simulink library "ECO_TestLibs"  (R2018a)
settings: Solver=ode45  StartTime=0.0  StopTime=10.0  RelTol=1e-3  EnableMultiTasking=on
undefined symbols (not defined in the file or in its folder): h, km
libraries: CoderSF_BSW_Libs x643, $bdroot x217, SF_CanService_Libs x60, simulink x12
(part 4 of 7)

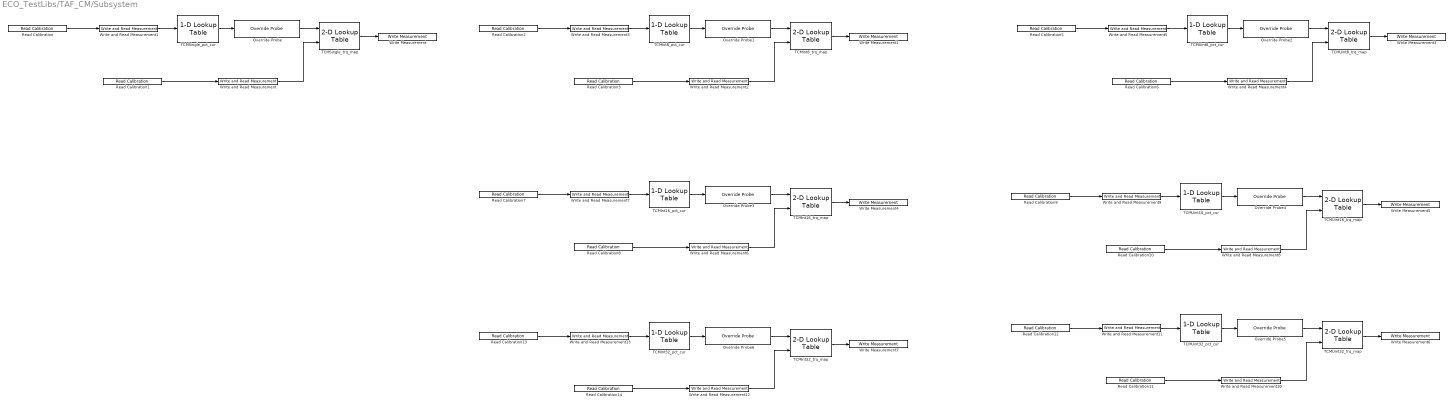
== system ECO_TestLibs/TAF_CM/Subsystem ==
  " Override Probe" : CoderSF_BSW_Libs/Calibration & Measurement/ Override Probe  variableName=TCMSingle_pct  variableValue=9  overrideValue=0  variableDataType=single  variableMin=[]  variableMax=[]  variableUnitStr=%
      settings: SourceProductName=EcoCoder Blocks
  " Override Probe1" : CoderSF_BSW_Libs/Calibration & Measurement/ Override Probe  variableName=TCMInt8_pct  variableValue=9  overrideValue=0  variableDataType=int8  variableMin=[]  variableMax=[]  variableUnitStr=%
      settings: SourceProductName=EcoCoder Blocks
  " Override Probe2" : CoderSF_BSW_Libs/Calibration & Measurement/ Override Probe  variableName=TCMUint8_pct  variableValue=9  overrideValue=0  variableDataType=uint8  variableMin=[]  variableMax=[]  variableUnitStr=%
      settings: SourceProductName=EcoCoder Blocks
  " Override Probe3" : CoderSF_BSW_Libs/Calibration & Measurement/ Override Probe  variableName=TCMInt16_pct  variableValue=9  overrideValue=0  variableDataType=int16  variableMin=[]  variableMax=[]  variableUnitStr=%
      settings: SourceProductName=EcoCoder Blocks
  " Override Probe4" : CoderSF_BSW_Libs/Calibration & Measurement/ Override Probe  variableName=TCMUint16_pct  variableValue=9  overrideValue=0  variableDataType=uint16  variableMin=[]  variableMax=[]  variableUnitStr=%
      settings: SourceProductName=EcoCoder Blocks
  " Override Probe5" : CoderSF_BSW_Libs/Calibration & Measurement/ Override Probe  variableName=TCMUint32_pct  variableValue=9  overrideValue=0  variableDataType=uint32  variableMin=[]  variableMax=[]  variableUnitStr=%
      settings: SourceProductName=EcoCoder Blocks
  " Override Probe6" : CoderSF_BSW_Libs/Calibration & Measurement/ Override Probe  variableName=TCMInt32_pct  variableValue=9  overrideValue=0  variableDataType=int32  variableMin=[]  variableMax=[]  variableUnitStr=%
      settings: SourceProductName=EcoCoder Blocks
  Read Calibration : CoderSF_BSW_Libs/Calibration & Measurement/Read Calibration  variable_name=TCMSingle_volt_val  variable_value=1  variable_type=single  variable_min=[]  variable_max=[]  unitStr=V  descStr=""
      settings: AttributesFormatString=value:%<variable_value> type:%<variable_type> max:%<variable_max> Min:%<variable_min>  SourceProductName=EcoCoder Blocks
  Read Calibration1 : CoderSF_BSW_Libs/Calibration & Measurement/Read Calibration  variable_name=TCMSingle_linspd_val  variable_value=20  variable_type=single  variable_min=[]  variable_max=[]  unitStr=km/h  descStr=""
      settings: AttributesFormatString=value:%<variable_value> type:%<variable_type> max:%<variable_max> Min:%<variable_min>  SourceProductName=EcoCoder Blocks
  Read Calibration10 : CoderSF_BSW_Libs/Calibration & Measurement/Read Calibration  variable_name=TCMUint16_linspd_val  variable_value=20  variable_type=uint16  variable_min=[]  variable_max=[]  unitStr=km/h  descStr=""
      settings: AttributesFormatString=value:%<variable_value> type:%<variable_type> max:%<variable_max> Min:%<variable_min>  SourceProductName=EcoCoder Blocks
  Read Calibration11 : CoderSF_BSW_Libs/Calibration & Measurement/Read Calibration  variable_name=TCMUint32_linspd_val  variable_value=20  variable_type=uint32  variable_min=[]  variable_max=[]  unitStr=km/h  descStr=""
      settings: AttributesFormatString=value:%<variable_value> type:%<variable_type> max:%<variable_max> Min:%<variable_min>  SourceProductName=EcoCoder Blocks
  Read Calibration12 : CoderSF_BSW_Libs/Calibration & Measurement/Read Calibration  variable_name=TCMUint32_volt_val  variable_value=1  variable_type=uint32  variable_min=[]  variable_max=[]  unitStr=V  descStr=""
      settings: AttributesFormatString=value:%<variable_value> type:%<variable_type> max:%<variable_max> Min:%<variable_min>  SourceProductName=EcoCoder Blocks
  Read Calibration13 : CoderSF_BSW_Libs/Calibration & Measurement/Read Calibration  variable_name=TCMInt32_volt_val  variable_value=1  variable_type=int32  variable_min=[]  variable_max=[]  unitStr=V  descStr=""
      settings: AttributesFormatString=value:%<variable_value> type:%<variable_type> max:%<variable_max> Min:%<variable_min>  SourceProductName=EcoCoder Blocks
  Read Calibration14 : CoderSF_BSW_Libs/Calibration & Measurement/Read Calibration  variable_name=TCMInt32_linspd_val  variable_value=20  variable_type=int32  variable_min=[]  variable_max=[]  unitStr=km/h  descStr=""
      settings: AttributesFormatString=value:%<variable_value> type:%<variable_type> max:%<variable_max> Min:%<variable_min>  SourceProductName=EcoCoder Blocks
  Read Calibration2 : CoderSF_BSW_Libs/Calibration & Measurement/Read Calibration  variable_name=TCMInt8_volt_val  variable_value=1  variable_type=int8  variable_min=[]  variable_max=[]  unitStr=V  descStr=""
      settings: AttributesFormatString=value:%<variable_value> type:%<variable_type> max:%<variable_max> Min:%<variable_min>  SourceProductName=EcoCoder Blocks
  Read Calibration3 : CoderSF_BSW_Libs/Calibration & Measurement/Read Calibration  variable_name=TCMInt8_linspd_val  variable_value=20  variable_type=int8  variable_min=[]  variable_max=[]  unitStr=km/h  descStr=""
      settings: AttributesFormatString=value:%<variable_value> type:%<variable_type> max:%<variable_max> Min:%<variable_min>  SourceProductName=EcoCoder Blocks
  Read Calibration5 : CoderSF_BSW_Libs/Calibration & Measurement/Read Calibration  variable_name=TCMUint8_volt_val  variable_value=1  variable_type=uint8  variable_min=[]  variable_max=[]  unitStr=V  descStr=""
      settings: AttributesFormatString=value:%<variable_value> type:%<variable_type> max:%<variable_max> Min:%<variable_min>  SourceProductName=EcoCoder Blocks
  Read Calibration6 : CoderSF_BSW_Libs/Calibration & Measurement/Read Calibration  variable_name=TCMUint8_linspd_val  variable_value=20  variable_type=uint8  variable_min=[]  variable_max=[]  unitStr=km/h  descStr=""
      settings: AttributesFormatString=value:%<variable_value> type:%<variable_type> max:%<variable_max> Min:%<variable_min>  SourceProductName=EcoCoder Blocks
  Read Calibration7 : CoderSF_BSW_Libs/Calibration & Measurement/Read Calibration  variable_name=TCMInt16_volt_val  variable_value=1  variable_type=int16  variable_min=[]  variable_max=[]  unitStr=V  descStr=""
      settings: AttributesFormatString=value:%<variable_value> type:%<variable_type> max:%<variable_max> Min:%<variable_min>  SourceProductName=EcoCoder Blocks
  Read Calibration8 : CoderSF_BSW_Libs/Calibration & Measurement/Read Calibration  variable_name=TCMInt16_linspd_val  variable_value=20  variable_type=int16  variable_min=[]  variable_max=[]  unitStr=km/h  descStr=""
      settings: AttributesFormatString=value:%<variable_value> type:%<variable_type> max:%<variable_max> Min:%<variable_min>  SourceProductName=EcoCoder Blocks
  Read Calibration9 : CoderSF_BSW_Libs/Calibration & Measurement/Read Calibration  variable_name=TCMUint16_volt_val  variable_value=1  variable_type=uint16  variable_min=[]  variable_max=[]  unitStr=V  descStr=""
      settings: AttributesFormatString=value:%<variable_value> type:%<variable_type> max:%<variable_max> Min:%<variable_min>  SourceProductName=EcoCoder Blocks
  TCMInt16_pct_cur : CoderSF_BSW_Libs/Calibration & Measurement/1-D Lookup Table  nam=TCMInt16_pct  breakpoint_type=int16  breakpoint_data=[0 5]  table_type=int16  table_data=[0 100]
      settings: SourceProductName=EcoCoder Blocks
  TCMInt16_trq_map : CoderSF_BSW_Libs/Calibration & Measurement/2-D Lookup Table  nam=TCMInt16_trq  breakpoint1_type=int16  breakpoint1_data=[0 50 100]  breakpoint2_type=int16  breakpoint2_data=[0 40 80 120]  table_type=int16  table_data=[20 40 40 30 ;20 50 40 30;20 40 50 80]
      settings: SourceProductName=EcoCoder Blocks
  TCMInt32_pct_cur : CoderSF_BSW_Libs/Calibration & Measurement/1-D Lookup Table  nam=TCMInt32_pct  breakpoint_type=int32  breakpoint_data=[0 5]  table_type=int32  table_data=[0 100]
      settings: SourceProductName=EcoCoder Blocks
  TCMInt32_trq_map : CoderSF_BSW_Libs/Calibration & Measurement/2-D Lookup Table  nam=TCMInt32_trq  breakpoint1_type=int32  breakpoint1_data=[0 50 100]  breakpoint2_type=int32  breakpoint2_data=[0 40 80 120]  table_type=int32  table_data=[20 40 40 30 ;20 50 40 30;20 40 50 80]
      settings: SourceProductName=EcoCoder Blocks
  TCMInt8_pct_cur : CoderSF_BSW_Libs/Calibration & Measurement/1-D Lookup Table  nam=TCMInt8_pct  breakpoint_type=int8  breakpoint_data=[0 5]  table_type=int8  table_data=[0 100]
      settings: SourceProductName=EcoCoder Blocks
  TCMInt8_trq_map : CoderSF_BSW_Libs/Calibration & Measurement/2-D Lookup Table  nam=TCMInt8_trq  breakpoint1_type=int8  breakpoint1_data=[0 50 100]  breakpoint2_type=int8  breakpoint2_data=[0 40 80 120]  table_type=int8  table_data=[20 40 40 30 ;20 50 40 30;20 40 50 80]
      settings: SourceProductName=EcoCoder Blocks
  TCMSingle_pct_cur : CoderSF_BSW_Libs/Calibration & Measurement/1-D Lookup Table  nam=TCMSingle_pct  breakpoint_type=single  breakpoint_data=[0 5]  table_type=single  table_data=[0 100]
      settings: SourceProductName=EcoCoder Blocks
  TCMSingle_trq_map : CoderSF_BSW_Libs/Calibration & Measurement/2-D Lookup Table  nam=TCMSingle_trq  breakpoint1_type=single  breakpoint1_data=[0 50 100]  breakpoint2_type=single  breakpoint2_data=[0 40 80 120]  table_type=single  table_data=[20 40 40 30 ;20 50 40 30;20 40 50 80]
      settings: SourceProductName=EcoCoder Blocks
  TCMUint16_pct_cur : CoderSF_BSW_Libs/Calibration & Measurement/1-D Lookup Table  nam=TCMUint16_pct  breakpoint_type=uint16  breakpoint_data=[0 5]  table_type=uint16  table_data=[0 100]
      settings: SourceProductName=EcoCoder Blocks
  TCMUint16_trq_map : CoderSF_BSW_Libs/Calibration & Measurement/2-D Lookup Table  nam=TCMUint16_trq  breakpoint1_type=uint16  breakpoint1_data=[0 50 100]  breakpoint2_type=uint16  breakpoint2_data=[0 40 80 120]  table_type=uint16  table_data=[20 40 40 30 ;20 50 40 30;20 40 50 80]
      settings: SourceProductName=EcoCoder Blocks
  TCMUint32_pct_cur : CoderSF_BSW_Libs/Calibration & Measurement/1-D Lookup Table  nam=TCMUint32_pct  breakpoint_type=uint32  breakpoint_data=[0 5]  table_type=uint32  table_data=[0 100]
      settings: SourceProductName=EcoCoder Blocks
  TCMUint32_trq_map : CoderSF_BSW_Libs/Calibration & Measurement/2-D Lookup Table  nam=TCMUint32_trq  breakpoint1_type=uint32  breakpoint1_data=[0 50 100]  breakpoint2_type=uint32  breakpoint2_data=[0 40 80 120]  table_type=uint32  table_data=[20 40 40 30 ;20 50 40 30;20 40 50 80]
      settings: SourceProductName=EcoCoder Blocks
  TCMUint8_pct_cur : CoderSF_BSW_Libs/Calibration & Measurement/1-D Lookup Table  nam=TCMUint8_pct  breakpoint_type=uint8  breakpoint_data=[0 5]  table_type=uint8  table_data=[0 100]
      settings: SourceProductName=EcoCoder Blocks
  TCMUint8_trq_map : CoderSF_BSW_Libs/Calibration & Measurement/2-D Lookup Table  nam=TCMUint8_trq  breakpoint1_type=uint8  breakpoint1_data=[0 50 100]  breakpoint2_type=uint8  breakpoint2_data=[0 40 80 120]  table_type=uint8  table_data=[20 40 40 30 ;20 50 40 30;20 40 50 80]
      settings: SourceProductName=EcoCoder Blocks
  Write Measurement : CoderSF_BSW_Libs/Calibration & Measurement/Write Measurement  variable_name=TCMSingle_trq  variable_value=0  variable_type=single  numD=1  unitStr=Nm  descStr=""
      settings: AttributesFormatString=value:%<variable_value> type:%<variable_type>  SourceProductName=EcoCoder Blocks
  Write Measurement1 : CoderSF_BSW_Libs/Calibration & Measurement/Write Measurement  variable_name=TCMInt8_trq  variable_value=0  variable_type=int8  numD=1  unitStr=Nm  descStr=""
      settings: AttributesFormatString=value:%<variable_value> type:%<variable_type>  SourceProductName=EcoCoder Blocks
  Write Measurement3 : CoderSF_BSW_Libs/Calibration & Measurement/Write Measurement  variable_name=TCMUint8_trq  variable_value=0  variable_type=uint8  numD=1  unitStr=Nm  descStr=""
      settings: AttributesFormatString=value:%<variable_value> type:%<variable_type>  SourceProductName=EcoCoder Blocks
  Write Measurement4 : CoderSF_BSW_Libs/Calibration & Measurement/Write Measurement  variable_name=TCMInt16_trq  variable_value=0  variable_type=int16  numD=1  unitStr=Nm  descStr=""
      settings: AttributesFormatString=value:%<variable_value> type:%<variable_type>  SourceProductName=EcoCoder Blocks
  Write Measurement5 : CoderSF_BSW_Libs/Calibration & Measurement/Write Measurement  variable_name=TCMUint16_trq  variable_value=0  variable_type=uint16  numD=1  unitStr=Nm  descStr=""
      settings: AttributesFormatString=value:%<variable_value> type:%<variable_type>  SourceProductName=EcoCoder Blocks
  Write Measurement6 : CoderSF_BSW_Libs/Calibration & Measurement/Write Measurement  variable_name=TCMUint32_trq  variable_value=0  variable_type=uint32  numD=1  unitStr=Nm  descStr=""
      settings: AttributesFormatString=value:%<variable_value> type:%<variable_type>  SourceProductName=EcoCoder Blocks
  Write Measurement7 : CoderSF_BSW_Libs/Calibration & Measurement/Write Measurement  variable_name=TCMInt32_trq  variable_value=0  variable_type=int32  numD=1  unitStr=Nm  descStr=""
      settings: AttributesFormatString=value:%<variable_value> type:%<variable_type>  SourceProductName=EcoCoder Blocks
  Write and Read Measurement : CoderSF_BSW_Libs/Calibration & Measurement/Write and Read Measurement  variable_name=TCMSingle_linspd  variable_value=0  variable_type=single  numD=1  unitStr=km/h  descStr=""
      settings: AttributesFormatString=value:%<variable_value> type:%<variable_type>  SourceProductName=EcoCoder Blocks
  Write and Read Measurement1 : CoderSF_BSW_Libs/Calibration & Measurement/Write and Read Measurement  variable_name=TCMSingle_volt  variable_value=0  variable_type=single  numD=1  unitStr=V  descStr=""
      settings: AttributesFormatString=value:%<variable_value> type:%<variable_type>  SourceProductName=EcoCoder Blocks
  Write and Read Measurement10 : CoderSF_BSW_Libs/Calibration & Measurement/Write and Read Measurement  variable_name=TCMUint32_linspd  variable_value=0  variable_type=uint32  numD=1  unitStr=km/h  descStr=""
      settings: AttributesFormatString=value:%<variable_value> type:%<variable_type>  SourceProductName=EcoCoder Blocks
  Write and Read Measurement11 : CoderSF_BSW_Libs/Calibration & Measurement/Write and Read Measurement  variable_name=TCMUint32_volt  variable_value=0  variable_type=uint32  numD=1  unitStr=V  descStr=""
      settings: AttributesFormatString=value:%<variable_value> type:%<variable_type>  SourceProductName=EcoCoder Blocks
  Write and Read Measurement12 : CoderSF_BSW_Libs/Calibration & Measurement/Write and Read Measurement  variable_name=TCMInt32_linspd  variable_value=0  variable_type=int32  numD=1  unitStr=km/h  descStr=""
      settings: AttributesFormatString=value:%<variable_value> type:%<variable_type>  SourceProductName=EcoCoder Blocks
  Write and Read Measurement13 : CoderSF_BSW_Libs/Calibration & Measurement/Write and Read Measurement  variable_name=TCMInt32_volt  variable_value=0  variable_type=int32  numD=1  unitStr=V  descStr=""
      settings: AttributesFormatString=value:%<variable_value> type:%<variable_type>  SourceProductName=EcoCoder Blocks
  Write and Read Measurement2 : CoderSF_BSW_Libs/Calibration & Measurement/Write and Read Measurement  variable_name=TCMInt8_linspd  variable_value=0  variable_type=int8  numD=1  unitStr=km/h  descStr=""
      settings: AttributesFormatString=value:%<variable_value> type:%<variable_type>  SourceProductName=EcoCoder Blocks
  Write and Read Measurement3 : CoderSF_BSW_Libs/Calibration & Measurement/Write and Read Measurement  variable_name=TCMInt8_volt  variable_value=0  variable_type=int8  numD=1  unitStr=V  descStr=""
      settings: AttributesFormatString=value:%<variable_value> type:%<variable_type>  SourceProductName=EcoCoder Blocks
  Write and Read Measurement4 : CoderSF_BSW_Libs/Calibration & Measurement/Write and Read Measurement  variable_name=TCMUint8_linspd  variable_value=0  variable_type=uint8  numD=1  unitStr=km/h  descStr=""
      settings: AttributesFormatString=value:%<variable_value> type:%<variable_type>  SourceProductName=EcoCoder Blocks
  Write and Read Measurement5 : CoderSF_BSW_Libs/Calibration & Measurement/Write and Read Measurement  variable_name=TCMUint8_volt  variable_value=0  variable_type=uint8  numD=1  unitStr=V  descStr=""
      settings: AttributesFormatString=value:%<variable_value> type:%<variable_type>  SourceProductName=EcoCoder Blocks
  Write and Read Measurement6 : CoderSF_BSW_Libs/Calibration & Measurement/Write and Read Measurement  variable_name=TCMInt16_linspd  variable_value=0  variable_type=int16  numD=1  unitStr=km/h  descStr=""
      settings: AttributesFormatString=value:%<variable_value> type:%<variable_type>  SourceProductName=EcoCoder Blocks
  Write and Read Measurement7 : CoderSF_BSW_Libs/Calibration & Measurement/Write and Read Measurement  variable_name=TCMInt16_volt  variable_value=0  variable_type=int16  numD=1  unitStr=V  descStr=""
      settings: AttributesFormatString=value:%<variable_value> type:%<variable_type>  SourceProductName=EcoCoder Blocks
  Write and Read Measurement8 : CoderSF_BSW_Libs/Calibration & Measurement/Write and Read Measurement  variable_name=TCMUint16_linspd  variable_value=0  variable_type=uint16  numD=1  unitStr=km/h  descStr=""
      settings: AttributesFormatString=value:%<variable_value> type:%<variable_type>  SourceProductName=EcoCoder Blocks
  Write and Read Measurement9 : CoderSF_BSW_Libs/Calibration & Measurement/Write and Read Measurement  variable_name=TCMUint16_volt  variable_value=0  variable_type=uint16  numD=1  unitStr=V  descStr=""
      settings: AttributesFormatString=value:%<variable_value> type:%<variable_type>  SourceProductName=EcoCoder Blocks
  wires:
  Read Calibration12/1 -> Write and Read Measurement11/1
  TCMUint32_pct_cur/1 -> " Override Probe5"/1
  Read Calibration/1 -> Write and Read Measurement1/1
  " Override Probe"/1 -> TCMSingle_trq_map/1
  TCMSingle_pct_cur/1 -> " Override Probe"/1
  Write and Read Measurement/1 -> TCMSingle_trq_map/2
  Write and Read Measurement1/1 -> TCMSingle_pct_cur/1
  TCMSingle_trq_map/1 -> Write Measurement/1
  Read Calibration1/1 -> Write and Read Measurement/1
  Read Calibration2/1 -> Write and Read Measurement3/1
  TCMInt8_pct_cur/1 -> " Override Probe1"/1
  " Override Probe1"/1 -> TCMInt8_trq_map/1
  Write and Read Measurement2/1 -> TCMInt8_trq_map/2
  Read Calibration3/1 -> Write and Read Measurement2/1
  TCMInt8_trq_map/1 -> Write Measurement1/1
  Write and Read Measurement3/1 -> TCMInt8_pct_cur/1
  Read Calibration5/1 -> Write and Read Measurement5/1
  TCMUint8_pct_cur/1 -> " Override Probe2"/1
  " Override Probe2"/1 -> TCMUint8_trq_map/1
  Write and Read Measurement4/1 -> TCMUint8_trq_map/2
  Read Calibration9/1 -> Write and Read Measurement9/1
  Write and Read Measurement6/1 -> TCMInt16_trq_map/2
  TCMInt16_trq_map/1 -> Write Measurement4/1
  Read Calibration6/1 -> Write and Read Measurement4/1
  Read Calibration8/1 -> Write and Read Measurement6/1
  TCMUint16_trq_map/1 -> Write Measurement5/1
  Write and Read Measurement5/1 -> TCMUint8_pct_cur/1
  Read Calibration7/1 -> Write and Read Measurement7/1
  " Override Probe4"/1 -> TCMUint16_trq_map/1
  TCMUint16_pct_cur/1 -> " Override Probe4"/1
  Write and Read Measurement8/1 -> TCMUint16_trq_map/2
  Write and Read Measurement7/1 -> TCMInt16_pct_cur/1
  TCMUint8_trq_map/1 -> Write Measurement3/1
  " Override Probe3"/1 -> TCMInt16_trq_map/1
  Write and Read Measurement9/1 -> TCMUint16_pct_cur/1
  Read Calibration10/1 -> Write and Read Measurement8/1
  TCMInt16_pct_cur/1 -> " Override Probe3"/1
  Write and Read Measurement13/1 -> TCMInt32_pct_cur/1
  Read Calibration14/1 -> Write and Read Measurement12/1
  TCMInt32_trq_map/1 -> Write Measurement7/1
  Write and Read Measurement12/1 -> TCMInt32_trq_map/2
  " Override Probe6"/1 -> TCMInt32_trq_map/1
  TCMInt32_pct_cur/1 -> " Override Probe6"/1
  Read Calibration13/1 -> Write and Read Measurement13/1
  Write and Read Measurement11/1 -> TCMUint32_pct_cur/1
  Read Calibration11/1 -> Write and Read Measurement10/1
  TCMUint32_trq_map/1 -> Write Measurement6/1
  Write and Read Measurement10/1 -> TCMUint32_trq_map/2
  " Override Probe5"/1 -> TCMUint32_trq_map/1

== system ECO_TestLibs/TAF_CM/TAF_DataByAddr ==
  Enable : EnablePort
  Calibration Definition : CoderSF_BSW_Libs/Calibration & Measurement/Calibration Definition  variable_name=DataReadDialog_addr_val  variable_value=hex2dec('00018100')  variable_type=uint32  variable_min=[]  variable_max=[]  unitStr=""  descStr=""
      settings: AttributesFormatString=value:%<variable_value> type:%<variable_type> max:%<variable_max> Min:%<variable_min>  SourceProductName=EcoCoder Blocks
  Read Calibration : CoderSF_BSW_Libs/Calibration & Measurement/Read Calibration  variable_name=DataRead_addr_val  variable_value=hex2dec('00018100')  variable_type=uint32  variable_min=[]  variable_max=[]  unitStr=""  descStr=""
      settings: AttributesFormatString=value:%<variable_value> type:%<variable_type> max:%<variable_max> Min:%<variable_min>  SourceProductName=EcoCoder Blocks
  Read Data By Address(Input port) : CoderSF_BSW_Libs/Advanced Data Blocks/Read Data By Address(Input port)  Len=8
      settings: SourceProductName=EcoCoder Blocks
  Read Data By Address1 : CoderSF_BSW_Libs/Advanced Data Blocks/Read Data By Address  Len=8  Offset=DataReadDialog_addr_val
      settings: SourceProductName=EcoCoder Blocks
  Write Measurement : CoderSF_BSW_Libs/Calibration & Measurement/Write Measurement  variable_name=DataRead_data  variable_value=0  variable_type=uint8  numD=8  unitStr=""  descStr=""
      settings: AttributesFormatString=type:%<variable_type> Dimensions:%<numD>  SourceProductName=EcoCoder Blocks
  Write Measurement4 : CoderSF_BSW_Libs/Calibration & Measurement/Write Measurement  variable_name=DataReadDialog_data  variable_value=0  variable_type=uint8  numD=8  unitStr=""  descStr=""
      settings: AttributesFormatString=type:%<variable_type> Dimensions:%<numD>  SourceProductName=EcoCoder Blocks
  wires:
  Read Data By Address1/1 -> Write Measurement4/1
  Read Data By Address(Input port)/1 -> Write Measurement/1
  Read Calibration/1 -> Read Data By Address(Input port)/1

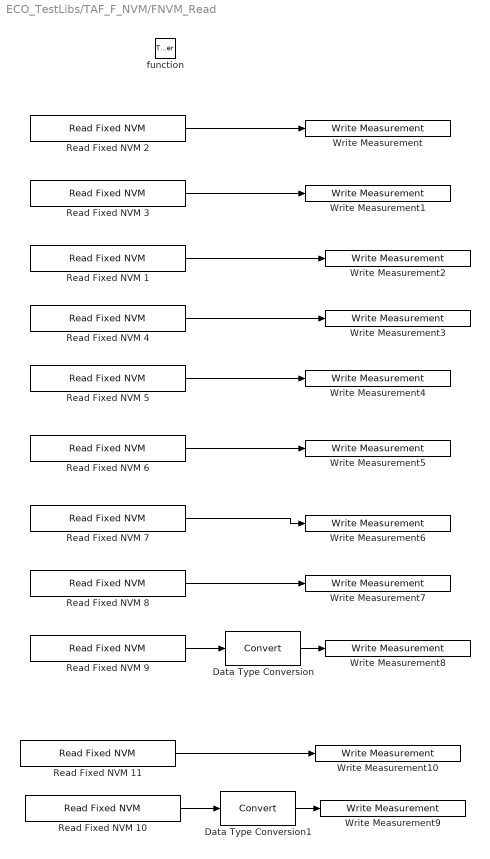
== system ECO_TestLibs/TAF_F_NVM/FNVM_Read ==
  function : TriggerPort  TriggerType=function-call  VariantControl=(inherit)
  Data Type Conversion : DataTypeConversion
  Data Type Conversion1 : DataTypeConversion
  Read Fixed NVM 1 : CoderSF_BSW_Libs/Non-volatile Memory Blocks/Read Fixed NVM   data_name=Fnvm_single
      settings: SourceProductName=EcoCoder Blocks
  Read Fixed NVM 10 : CoderSF_BSW_Libs/Non-volatile Memory Blocks/Read Fixed NVM   data_name=Fnvm_double2
      settings: SourceProductName=EcoCoder Blocks
  Read Fixed NVM 11 : CoderSF_BSW_Libs/Non-volatile Memory Blocks/Read Fixed NVM   data_name=Fnvm_single2
      settings: SourceProductName=EcoCoder Blocks
  Read Fixed NVM 2 : CoderSF_BSW_Libs/Non-volatile Memory Blocks/Read Fixed NVM   data_name=Fnvm_int32
      settings: SourceProductName=EcoCoder Blocks
  Read Fixed NVM 3 : CoderSF_BSW_Libs/Non-volatile Memory Blocks/Read Fixed NVM   data_name=Fnvm_uint32
      settings: SourceProductName=EcoCoder Blocks
  Read Fixed NVM 4 : CoderSF_BSW_Libs/Non-volatile Memory Blocks/Read Fixed NVM   data_name=Fnvm_int16
      settings: SourceProductName=EcoCoder Blocks
  Read Fixed NVM 5 : CoderSF_BSW_Libs/Non-volatile Memory Blocks/Read Fixed NVM   data_name=Fnvm_uint16
      settings: SourceProductName=EcoCoder Blocks
  Read Fixed NVM 6 : CoderSF_BSW_Libs/Non-volatile Memory Blocks/Read Fixed NVM   data_name=Fnvm_boolean
      settings: SourceProductName=EcoCoder Blocks
  Read Fixed NVM 7 : CoderSF_BSW_Libs/Non-volatile Memory Blocks/Read Fixed NVM   data_name=Fnvm_uint8
      settings: SourceProductName=EcoCoder Blocks
  Read Fixed NVM 8 : CoderSF_BSW_Libs/Non-volatile Memory Blocks/Read Fixed NVM   data_name=Fnvm_int8
      settings: SourceProductName=EcoCoder Blocks
  Read Fixed NVM 9 : CoderSF_BSW_Libs/Non-volatile Memory Blocks/Read Fixed NVM   data_name=Fnvm_double
      settings: SourceProductName=EcoCoder Blocks
  Write Measurement : CoderSF_BSW_Libs/Calibration & Measurement/Write Measurement  variable_name=Fnvm_int32_v  variable_value=0  variable_type=int32  numD=1  unitStr=""  descStr=""
      settings: AttributesFormatString=value:%<variable_value> type:%<variable_type>  SourceProductName=EcoCoder Blocks
  Write Measurement1 : CoderSF_BSW_Libs/Calibration & Measurement/Write Measurement  variable_name=Fnvm_uint32_v  variable_value=0  variable_type=uint32  numD=4  unitStr=""  descStr=""
      settings: AttributesFormatString=value:%<variable_value> type:%<variable_type>  SourceProductName=EcoCoder Blocks
  Write Measurement10 : CoderSF_BSW_Libs/Calibration & Measurement/Write Measurement  variable_name=Fnvm_single2_v  variable_value=0  variable_type=single  numD=1  unitStr=""  descStr=""
      settings: AttributesFormatString=value:%<variable_value> type:%<variable_type>  SourceProductName=EcoCoder Blocks
  Write Measurement2 : CoderSF_BSW_Libs/Calibration & Measurement/Write Measurement  variable_name=Fnvm_single_v  variable_value=0  variable_type=single  numD=1  unitStr=""  descStr=""
      settings: AttributesFormatString=value:%<variable_value> type:%<variable_type>  SourceProductName=EcoCoder Blocks
  Write Measurement3 : CoderSF_BSW_Libs/Calibration & Measurement/Write Measurement  variable_name=Fnvm_int16_v  variable_value=0  variable_type=int16  numD=2  unitStr=""  descStr=""
      settings: AttributesFormatString=value:%<variable_value> type:%<variable_type>  SourceProductName=EcoCoder Blocks
  Write Measurement4 : CoderSF_BSW_Libs/Calibration & Measurement/Write Measurement  variable_name=Fnvm_uint16_v  variable_value=0  variable_type=uint16  numD=2  unitStr=""  descStr=""
      settings: AttributesFormatString=value:%<variable_value> type:%<variable_type>  SourceProductName=EcoCoder Blocks
  Write Measurement5 : CoderSF_BSW_Libs/Calibration & Measurement/Write Measurement  variable_name=Fnvm_boolean_v  variable_value=0  variable_type=boolean  numD=4  unitStr=""  descStr=""
      settings: AttributesFormatString=value:%<variable_value> type:%<variable_type>  SourceProductName=EcoCoder Blocks
  Write Measurement6 : CoderSF_BSW_Libs/Calibration & Measurement/Write Measurement  variable_name=Fnvm_uint8_v  variable_value=0  variable_type=uint8  numD=1  unitStr=""  descStr=""
      settings: AttributesFormatString=value:%<variable_value> type:%<variable_type>  SourceProductName=EcoCoder Blocks
  Write Measurement7 : CoderSF_BSW_Libs/Calibration & Measurement/Write Measurement  variable_name=Fnvm_int8_v  variable_value=0  variable_type=int8  numD=2  unitStr=""  descStr=""
      settings: AttributesFormatString=value:%<variable_value> type:%<variable_type>  SourceProductName=EcoCoder Blocks
  Write Measurement8 : CoderSF_BSW_Libs/Calibration & Measurement/Write Measurement  variable_name=Fnvm_double_v  variable_value=0  variable_type=single  numD=1  unitStr=""  descStr=""
      settings: AttributesFormatString=value:%<variable_value> type:%<variable_type>  SourceProductName=EcoCoder Blocks
  Write Measurement9 : CoderSF_BSW_Libs/Calibration & Measurement/Write Measurement  variable_name=Fnvm_double2_v  variable_value=0  variable_type=single  numD=1  unitStr=""  descStr=""
      settings: AttributesFormatString=value:%<variable_value> type:%<variable_type>  SourceProductName=EcoCoder Blocks
  wires:
  Read Fixed NVM 2/1 -> Write Measurement/1
  Read Fixed NVM 3/1 -> Write Measurement1/1
  Read Fixed NVM 1/1 -> Write Measurement2/1
  Read Fixed NVM 4/1 -> Write Measurement3/1
  Read Fixed NVM 5/1 -> Write Measurement4/1
  Read Fixed NVM 6/1 -> Write Measurement5/1
  Read Fixed NVM 7/1 -> Write Measurement6/1
  Read Fixed NVM 8/1 -> Write Measurement7/1
  Read Fixed NVM 9/1 -> Data Type Conversion/1
  Data Type Conversion/1 -> Write Measurement8/1
  Read Fixed NVM 10/1 -> Data Type Conversion1/1
  Data Type Conversion1/1 -> Write Measurement9/1
  Read Fixed NVM 11/1 -> Write Measurement10/1

== system ECO_TestLibs/TAF_F_NVM/FNVM_ReadAndWrite ==
  FNVM_ReadAndWrite : Subsystem
      settings: AttributesFormatString=%<Priority>
  Task_Call3 : CoderSF_BSW_Libs/Task Scheduler/Task Trigger  tasktimeIndex=Task_ini
      settings: SourceProductName=EcoCoder Blocks
  wires:
  Task_Call3/1 -> FNVM_ReadAndWrite/Trigger

== system ECO_TestLibs/TAF_F_NVM/FNVM_ReadBeforeWrite ==
  FNVM_ReadBeforeWrite : Subsystem
      settings: AttributesFormatString=%<Priority>
  Task_Call2 : CoderSF_BSW_Libs/Task Scheduler/Task Trigger  tasktimeIndex=Task_ini
      settings: SourceProductName=EcoCoder Blocks
  wires:
  Task_Call2/1 -> FNVM_ReadBeforeWrite/Trigger

== system ECO_TestLibs/TAF_NF_NVM/NVM_Read ==
  function : TriggerPort  TriggerType=function-call  VariantControl=(inherit)
  Measurement Probe : CoderSF_BSW_Libs/Calibration & Measurement/Write Measurement  variable_name=ASW_V_single  variable_value=0  variable_type=single  numD=1  unitStr=""  descStr=""
      settings: AttributesFormatString=value:%<variable_value> type:%<variable_type>  SourceProductName=EcoCoder Blocks
  Measurement Probe1 : CoderSF_BSW_Libs/Calibration & Measurement/Write Measurement  variable_name=ASW_V_int8  variable_value=0  variable_type=int8  numD=1  unitStr=""  descStr=""
      settings: AttributesFormatString=value:%<variable_value> type:%<variable_type>  SourceProductName=EcoCoder Blocks
  Measurement Probe2 : CoderSF_BSW_Libs/Calibration & Measurement/Write Measurement  variable_name=ASW_V_uint8  variable_value=0  variable_type=uint8  numD=1  unitStr=""  descStr=""
      settings: AttributesFormatString=value:%<variable_value> type:%<variable_type>  SourceProductName=EcoCoder Blocks
  Measurement Probe3 : CoderSF_BSW_Libs/Calibration & Measurement/Write Measurement  variable_name=ASW_V_int16  variable_value=0  variable_type=int16  numD=1  unitStr=""  descStr=""
      settings: AttributesFormatString=value:%<variable_value> type:%<variable_type>  SourceProductName=EcoCoder Blocks
  Measurement Probe4 : CoderSF_BSW_Libs/Calibration & Measurement/Write Measurement  variable_name=ASW_V_uint16  variable_value=0  variable_type=uint16  numD=1  unitStr=""  descStr=""
      settings: AttributesFormatString=value:%<variable_value> type:%<variable_type>  SourceProductName=EcoCoder Blocks
  Measurement Probe5 : CoderSF_BSW_Libs/Calibration & Measurement/Write Measurement  variable_name=ASW_V_int32  variable_value=0  variable_type=int32  numD=1  unitStr=""  descStr=""
      settings: AttributesFormatString=value:%<variable_value> type:%<variable_type>  SourceProductName=EcoCoder Blocks
  Measurement Probe6 : CoderSF_BSW_Libs/Calibration & Measurement/Write Measurement  variable_name=ASW_V_uint32  variable_value=0  variable_type=uint32  numD=1  unitStr=""  descStr=""
      settings: AttributesFormatString=value:%<variable_value> type:%<variable_type>  SourceProductName=EcoCoder Blocks
  Measurement Probe7 : CoderSF_BSW_Libs/Calibration & Measurement/Write Measurement  variable_name=ASW_V_boolean  variable_value=0  variable_type=boolean  numD=1  unitStr=""  descStr=""
      settings: AttributesFormatString=value:%<variable_value> type:%<variable_type>  SourceProductName=EcoCoder Blocks
  Read Nvmem : CoderSF_BSW_Libs/Non-volatile Memory Blocks/Read NVM  variable_name=ASW_Nvm_single  variable_type=Inherit from 'Variable definition'
      settings: AttributesFormatString=type:%<variable_type>  SourceProductName=EcoCoder Blocks
  Read Nvmem1 : CoderSF_BSW_Libs/Non-volatile Memory Blocks/Read NVM  variable_name=ASW_Nvm_int8  variable_type=Inherit from 'Variable definition'
      settings: AttributesFormatString=type:%<variable_type>  SourceProductName=EcoCoder Blocks
  Read Nvmem2 : CoderSF_BSW_Libs/Non-volatile Memory Blocks/Read NVM  variable_name=ASW_Nvm_uint8  variable_type=Inherit from 'Variable definition'
      settings: AttributesFormatString=type:%<variable_type>  SourceProductName=EcoCoder Blocks
  Read Nvmem3 : CoderSF_BSW_Libs/Non-volatile Memory Blocks/Read NVM  variable_name=ASW_Nvm_int16  variable_type=Inherit from 'Variable definition'
      settings: AttributesFormatString=type:%<variable_type>  SourceProductName=EcoCoder Blocks
  Read Nvmem4 : CoderSF_BSW_Libs/Non-volatile Memory Blocks/Read NVM  variable_name=ASW_Nvm_uint16  variable_type=Inherit from 'Variable definition'
      settings: AttributesFormatString=type:%<variable_type>  SourceProductName=EcoCoder Blocks
  Read Nvmem5 : CoderSF_BSW_Libs/Non-volatile Memory Blocks/Read NVM  variable_name=ASW_Nvm_int32  variable_type=Inherit from 'Variable definition'
      settings: AttributesFormatString=type:%<variable_type>  SourceProductName=EcoCoder Blocks
  Read Nvmem6 : CoderSF_BSW_Libs/Non-volatile Memory Blocks/Read NVM  variable_name=ASW_Nvm_uint32  variable_type=Inherit from 'Variable definition'
      settings: AttributesFormatString=type:%<variable_type>  SourceProductName=EcoCoder Blocks
  Read Nvmem7 : CoderSF_BSW_Libs/Non-volatile Memory Blocks/Read NVM  variable_name=ASW_Nvm_boolean  variable_type=Inherit from 'Variable definition'
      settings: AttributesFormatString=type:%<variable_type>  SourceProductName=EcoCoder Blocks
  wires:
  Read Nvmem/1 -> Measurement Probe/1
  Read Nvmem1/1 -> Measurement Probe1/1
  Read Nvmem2/1 -> Measurement Probe2/1
  Read Nvmem3/1 -> Measurement Probe3/1
  Read Nvmem4/1 -> Measurement Probe4/1
  Read Nvmem5/1 -> Measurement Probe5/1
  Read Nvmem6/1 -> Measurement Probe6/1
  Read Nvmem7/1 -> Measurement Probe7/1

== system ECO_TestLibs/TAF_NF_NVM/NVM_ReadAndWrite ==
  NVM_ReadAndWrite : Subsystem
      settings: AttributesFormatString=%<Priority>
  Task_Call3 : CoderSF_BSW_Libs/Task Scheduler/Task Trigger  tasktimeIndex=Task_ini
      settings: SourceProductName=EcoCoder Blocks
  wires:
  Task_Call3/1 -> NVM_ReadAndWrite/Trigger

== system ECO_TestLibs/TAF_NF_NVM/NVM_ReadBeforeWrite ==
  NVM_ReadBeforeWrite : Subsystem
      settings: AttributesFormatString=%<Priority>
  Task_Call2 : CoderSF_BSW_Libs/Task Scheduler/Task Trigger  tasktimeIndex=Task_ini
      settings: SourceProductName=EcoCoder Blocks
  wires:
  Task_Call2/1 -> NVM_ReadBeforeWrite/Trigger

== system ECO_TestLibs/TAF_NF_NVM/Test_NVMStoreFailed ==
  function : TriggerPort  TriggerType=function-call  VariantControl=(inherit)
  F_Store_All_NVM_Data : Subsystem  TreatAsAtomicUnit=on
      settings: RTWSystemCode=Nonreusable function  RTWFcnNameOpts=Use subsystem name
  While Function Only Code : S-Function  FunctionName=ecocoder_sf_while  SFunctionDeploymentMode=off  EnableBusSupport=off  mask(While Function Only Code){}
      mask help: While Function Only Code
      mask Display: disp('While Function Only Code');
  ecocoder_calibration : CoderSF_BSW_Libs/Calibration & Measurement/Read Calibration  variable_name=ASW_flgNVMStoreWhile_val  variable_value=0  variable_type=boolean  variable_min=[]  variable_max=[]  unitStr=""  descStr=""
      settings: AttributesFormatString=value:%<variable_value> type:%<variable_type> max:%<variable_max> Min:%<variable_min>  SourceProductName=EcoCoder Blocks
  ecocoder_measurement : CoderSF_BSW_Libs/Calibration & Measurement/Write and Read Measurement  variable_name=ASW_flgNVMStoreWhile  variable_value=0  variable_type=boolean  numD=1  unitStr=""  descStr=""
      settings: AttributesFormatString=value:%<variable_value> type:%<variable_type>  SourceProductName=EcoCoder Blocks
  wires:
  While Function Only Code/1 -> F_Store_All_NVM_Data/Trigger
  ecocoder_measurement/1 -> While Function Only Code/1
  ecocoder_calibration/1 -> ecocoder_measurement/1

== system ECO_TestLibs/TAF_SWD/TAF_SWD ==
  function : TriggerPort  TriggerType=function-call  VariantControl=(inherit)
  Service Software Watchdog : Subsystem  TreatAsAtomicUnit=on
      settings: RTWFcnNameOpts=Use subsystem name
  ecocoder_calibration : CoderSF_BSW_Libs/Calibration & Measurement/Read Calibration  variable_name=SY_flgSerDogEn_val  variable_value=1  variable_type=uint32  variable_min=[]  variable_max=[]  unitStr=""  descStr=""
      settings: AttributesFormatString=value:%<variable_value> type:%<variable_type> max:%<variable_max> Min:%<variable_min>  SourceProductName=EcoCoder Blocks
  wires:
  ecocoder_calibration/1 -> Service Software Watchdog/Enable

== system ECO_TestLibs/TAF_SYS/Function-Call Subsystem1 ==
  function : TriggerPort  TriggerType=function-call  VariantControl=(inherit)
  Read Calibration : CoderSF_BSW_Libs/Calibration & Measurement/Read Calibration  variable_name=TAF_SYS_datCANA_val  variable_value=[1 2 3 4 5 6 7 8]  variable_type=uint8  variable_min=[]  variable_max=[]  unitStr=""  descStr=""
      settings: AttributesFormatString=value:%<variable_value> type:%<variable_type> max:%<variable_max> Min:%<variable_min>  SourceProductName=EcoCoder Blocks
  Send CAN Data : CoderSF_BSW_Libs/CAN/Send CAN Data  channel=CAN_A  txlen=4  txid=hex2dec('111')  frametype=Standard(11-bit ID)  showerror=off
      settings: SourceProductName=EcoCoder Blocks
  Send CAN Data1 : CoderSF_BSW_Libs/CAN/Send CAN Data  channel=CAN_B  txlen=4  txid=hex2dec('112')  frametype=Standard(11-bit ID)  showerror=off
      settings: SourceProductName=EcoCoder Blocks
  Send CAN Data2 : CoderSF_BSW_Libs/CAN/Send CAN Data  channel=CAN_C  txlen=4  txid=hex2dec('113')  frametype=Standard(11-bit ID)  showerror=off
      settings: SourceProductName=EcoCoder Blocks
  wires:
  Read Calibration/1 -> Send CAN Data1/1, Send CAN Data2/1, Send CAN Data/1

== system ECO_TestLibs/TAF_SYS/Shutdown Power ==
  Enabled Subsystem : Subsystem  TreatAsAtomicUnit=on
  Read Calibration : CoderSF_BSW_Libs/Calibration & Measurement/Read Calibration  variable_name=WKUP_flgShtDwnHold_val  variable_value=0  variable_type=boolean  variable_min=[]  variable_max=[]  unitStr=""  descStr=""
      settings: AttributesFormatString=value:%<variable_value> type:%<variable_type> max:%<variable_max> Min:%<variable_min>  SourceProductName=EcoCoder Blocks
  Read Calibration1 : CoderSF_BSW_Libs/Calibration & Measurement/Read Calibration  variable_name=WKUP_flgShtDwnRising_val  variable_value=0  variable_type=boolean  variable_min=[]  variable_max=[]  unitStr=""  descStr=""
      settings: AttributesFormatString=value:%<variable_value> type:%<variable_type> max:%<variable_max> Min:%<variable_min>  SourceProductName=EcoCoder Blocks
  Read Calibration2 : CoderSF_BSW_Libs/Calibration & Measurement/Read Calibration  variable_name=WKUP_flgPwrDelaySet_val  variable_value=0  variable_type=boolean  variable_min=[]  variable_max=[]  unitStr=""  descStr=""
      settings: AttributesFormatString=value:%<variable_value> type:%<variable_type> max:%<variable_max> Min:%<variable_min>  SourceProductName=EcoCoder Blocks
  Shutdown Power : CoderSF_BSW_Libs/System Management Blocks/Shutdown Power  TriggerTypeSet=rising  tWait_ms=500
      settings: SourceProductName=EcoCoder Blocks
  Shutdown Power Hold : CoderSF_BSW_Libs/System Management Blocks/Shutdown Power Hold  tWait_ms=500
      settings: SourceProductName=EcoCoder Blocks
  Write and Read Measurement : CoderSF_BSW_Libs/Calibration & Measurement/Write and Read Measurement  variable_name=WKUP_flgShtDwnHold  variable_value=0  variable_type=boolean  numD=1  unitStr=""  descStr=""
      settings: AttributesFormatString=value:%<variable_value> type:%<variable_type>  SourceProductName=EcoCoder Blocks
  Write and Read Measurement1 : CoderSF_BSW_Libs/Calibration & Measurement/Write and Read Measurement  variable_name=WKUP_flgShtDwnRising  variable_value=0  variable_type=boolean  numD=1  unitStr=""  descStr=""
      settings: AttributesFormatString=value:%<variable_value> type:%<variable_type>  SourceProductName=EcoCoder Blocks
  wires:
  Read Calibration/1 -> Write and Read Measurement/1
  Write and Read Measurement/1 -> Shutdown Power Hold/Enable
  Read Calibration1/1 -> Write and Read Measurement1/1
  Write and Read Measurement1/1 -> Shutdown Power/Trigger
  Read Calibration2/1 -> Enabled Subsystem/Enable

== system ECO_TestLibs/TAF_SYS/Software Reset ==
  Read Calibration3 : CoderSF_BSW_Libs/Calibration & Measurement/Read Calibration  variable_name=WKUP_flgRestRising_val  variable_value=0  variable_type=boolean  variable_min=[]  variable_max=[]  unitStr=""  descStr=""
      settings: AttributesFormatString=value:%<variable_value> type:%<variable_type> max:%<variable_max> Min:%<variable_min>  SourceProductName=EcoCoder Blocks
  Read Calibration4 : CoderSF_BSW_Libs/Calibration & Measurement/Read Calibration  variable_name=WKUP_flgRestHold_val  variable_value=0  variable_type=boolean  variable_min=[]  variable_max=[]  unitStr=""  descStr=""
      settings: AttributesFormatString=value:%<variable_value> type:%<variable_type> max:%<variable_max> Min:%<variable_min>  SourceProductName=EcoCoder Blocks
  Software Reset : CoderSF_BSW_Libs/System Management Blocks/Software Reset  TriggerTypeSet=rising
      settings: SourceProductName=EcoCoder Blocks
  Software Reset Hold : CoderSF_BSW_Libs/System Management Blocks/Software Reset Hold
      settings: SourceProductName=EcoCoder Blocks
  Write and Read Measurement2 : CoderSF_BSW_Libs/Calibration & Measurement/Write and Read Measurement  variable_name=WKUP_flgRestRising  variable_value=0  variable_type=boolean  numD=1  unitStr=""  descStr=""
      settings: AttributesFormatString=value:%<variable_value> type:%<variable_type>  SourceProductName=EcoCoder Blocks
  Write and Read Measurement3 : CoderSF_BSW_Libs/Calibration & Measurement/Write and Read Measurement  variable_name=WKUP_flgRestHold  variable_value=0  variable_type=boolean  numD=1  unitStr=""  descStr=""
      settings: AttributesFormatString=value:%<variable_value> type:%<variable_type>  SourceProductName=EcoCoder Blocks
  wires:
  Read Calibration3/1 -> Write and Read Measurement2/1
  Write and Read Measurement2/1 -> Software Reset/Trigger
  Read Calibration4/1 -> Write and Read Measurement3/1
  Write and Read Measurement3/1 -> Software Reset Hold/Enable

== system ECO_TestLibs/TAF_TRI/FC_H10ms ==
  function : TriggerPort  TriggerType=function-call  VariantControl=(inherit)
  Display : Display
  GetPeriod_ms : $bdroot/GetPeriod_ms  frqP=TRI_frqFreeSys_val
  Write Measurement : CoderSF_BSW_Libs/Calibration & Measurement/Write Measurement  variable_name=TRI_tH10ms  variable_value=0  variable_type=single  numD=1  unitStr=ms  descStr=""
      settings: AttributesFormatString=value:%<variable_value> type:%<variable_type>  SourceProductName=EcoCoder Blocks
  dt : CoderSF_BSW_Libs/Application Base Blocks/dt
      settings: SourceProductName=EcoCoder Blocks
  wires:
  GetPeriod_ms/1 -> Write Measurement/1
  dt/1 -> Display/1

== system ECO_TestLibs/TAF_TRI/FC_H1ms ==
  function : TriggerPort  TriggerType=function-call  VariantControl=(inherit)
  Display : Display
  GetPeriod_ms : $bdroot/GetPeriod_ms  frqP=TRI_frqFreeSys_val
  Write Measurement : CoderSF_BSW_Libs/Calibration & Measurement/Write Measurement  variable_name=TRI_tH1ms  variable_value=0  variable_type=single  numD=1  unitStr=ms  descStr=""
      settings: AttributesFormatString=value:%<variable_value> type:%<variable_type>  SourceProductName=EcoCoder Blocks
  dt : CoderSF_BSW_Libs/Application Base Blocks/dt
      settings: SourceProductName=EcoCoder Blocks
  wires:
  GetPeriod_ms/1 -> Write Measurement/1
  dt/1 -> Display/1

== system ECO_TestLibs/TAF_TRI/FC_H20ms ==
  function : TriggerPort  TriggerType=function-call  VariantControl=(inherit)
  Display : Display
  GetPeriod_ms : $bdroot/GetPeriod_ms  frqP=TRI_frqFreeSys_val
  Write Measurement : CoderSF_BSW_Libs/Calibration & Measurement/Write Measurement  variable_name=TRI_tH20ms  variable_value=0  variable_type=single  numD=1  unitStr=ms  descStr=""
      settings: AttributesFormatString=value:%<variable_value> type:%<variable_type>  SourceProductName=EcoCoder Blocks
  dt : CoderSF_BSW_Libs/Application Base Blocks/dt
      settings: SourceProductName=EcoCoder Blocks
  wires:
  GetPeriod_ms/1 -> Write Measurement/1
  dt/1 -> Display/1

== system ECO_TestLibs/TAF_TRI/FC_H5ms ==
  function : TriggerPort  TriggerType=function-call  VariantControl=(inherit)
  Display : Display
  GetPeriod_ms : $bdroot/GetPeriod_ms  frqP=TRI_frqFreeSys_val
  Write Measurement : CoderSF_BSW_Libs/Calibration & Measurement/Write Measurement  variable_name=TRI_tH5ms  variable_value=0  variable_type=single  numD=1  unitStr=ms  descStr=""
      settings: AttributesFormatString=value:%<variable_value> type:%<variable_type>  SourceProductName=EcoCoder Blocks
  dt : CoderSF_BSW_Libs/Application Base Blocks/dt
      settings: SourceProductName=EcoCoder Blocks
  wires:
  GetPeriod_ms/1 -> Write Measurement/1
  dt/1 -> Display/1

== system ECO_TestLibs/TAF_TRI/FC_L1000ms ==
  function : TriggerPort  TriggerType=function-call  VariantControl=(inherit)
  Display : Display
  GetPeriod_ms : $bdroot/GetPeriod_ms  frqP=TRI_frqFreeSys_val
  Write Measurement : CoderSF_BSW_Libs/Calibration & Measurement/Write Measurement  variable_name=TRI_tL1000ms  variable_value=0  variable_type=single  numD=1  unitStr=ms  descStr=""
      settings: AttributesFormatString=value:%<variable_value> type:%<variable_type>  SourceProductName=EcoCoder Blocks
  dt : CoderSF_BSW_Libs/Application Base Blocks/dt
      settings: SourceProductName=EcoCoder Blocks
  wires:
  GetPeriod_ms/1 -> Write Measurement/1
  dt/1 -> Display/1

== system ECO_TestLibs/TAF_TRI/FC_L100ms ==
  function : TriggerPort  TriggerType=function-call  VariantControl=(inherit)
  Display : Display
  GetPeriod_ms : $bdroot/GetPeriod_ms  frqP=TRI_frqFreeSys_val
  Write Measurement : CoderSF_BSW_Libs/Calibration & Measurement/Write Measurement  variable_name=TRI_tL100ms  variable_value=0  variable_type=single  numD=1  unitStr=ms  descStr=""
      settings: AttributesFormatString=value:%<variable_value> type:%<variable_type>  SourceProductName=EcoCoder Blocks
  dt : CoderSF_BSW_Libs/Application Base Blocks/dt
      settings: SourceProductName=EcoCoder Blocks
  wires:
  GetPeriod_ms/1 -> Write Measurement/1
  dt/1 -> Display/1

== system ECO_TestLibs/TAF_TRI/FC_L10ms ==
  function : TriggerPort  TriggerType=function-call  VariantControl=(inherit)
  Display : Display
  GetPeriod_ms : $bdroot/GetPeriod_ms  frqP=TRI_frqFreeSys_val
  Write Measurement : CoderSF_BSW_Libs/Calibration & Measurement/Write Measurement  variable_name=TRI_tL10ms  variable_value=0  variable_type=single  numD=1  unitStr=ms  descStr=""
      settings: AttributesFormatString=value:%<variable_value> type:%<variable_type>  SourceProductName=EcoCoder Blocks
  dt : CoderSF_BSW_Libs/Application Base Blocks/dt
      settings: SourceProductName=EcoCoder Blocks
  wires:
  GetPeriod_ms/1 -> Write Measurement/1
  dt/1 -> Display/1

== system ECO_TestLibs/TAF_TRI/FC_L1ms ==
  function : TriggerPort  TriggerType=function-call  VariantControl=(inherit)
  Display : Display
  GetPeriod_ms : $bdroot/GetPeriod_ms  frqP=TRI_frqFreeSys_val
  Write Measurement : CoderSF_BSW_Libs/Calibration & Measurement/Write Measurement  variable_name=TRI_tL1ms  variable_value=0  variable_type=single  numD=1  unitStr=ms  descStr=""
      settings: AttributesFormatString=value:%<variable_value> type:%<variable_type>  SourceProductName=EcoCoder Blocks
  dt : CoderSF_BSW_Libs/Application Base Blocks/dt
      settings: SourceProductName=EcoCoder Blocks
  wires:
  GetPeriod_ms/1 -> Write Measurement/1
  dt/1 -> Display/1

== system ECO_TestLibs/TAF_TRI/FC_L200ms ==
  function : TriggerPort  TriggerType=function-call  VariantControl=(inherit)
  Display : Display
  GetPeriod_ms : $bdroot/GetPeriod_ms  frqP=TRI_frqFreeSys_val
  Write Measurement : CoderSF_BSW_Libs/Calibration & Measurement/Write Measurement  variable_name=TRI_tL200ms  variable_value=0  variable_type=single  numD=1  unitStr=ms  descStr=""
      settings: AttributesFormatString=value:%<variable_value> type:%<variable_type>  SourceProductName=EcoCoder Blocks
  dt : CoderSF_BSW_Libs/Application Base Blocks/dt
      settings: SourceProductName=EcoCoder Blocks
  wires:
  GetPeriod_ms/1 -> Write Measurement/1
  dt/1 -> Display/1

== system ECO_TestLibs/TAF_TRI/FC_L20ms ==
  function : TriggerPort  TriggerType=function-call  VariantControl=(inherit)
  Display : Display
  GetPeriod_ms : $bdroot/GetPeriod_ms  frqP=TRI_frqFreeSys_val
  Write Measurement : CoderSF_BSW_Libs/Calibration & Measurement/Write Measurement  variable_name=TRI_tL20ms  variable_value=0  variable_type=single  numD=1  unitStr=ms  descStr=""
      settings: AttributesFormatString=value:%<variable_value> type:%<variable_type>  SourceProductName=EcoCoder Blocks
  dt : CoderSF_BSW_Libs/Application Base Blocks/dt
      settings: SourceProductName=EcoCoder Blocks
  wires:
  GetPeriod_ms/1 -> Write Measurement/1
  dt/1 -> Display/1

== system ECO_TestLibs/TAF_TRI/FC_L500ms ==
  function : TriggerPort  TriggerType=function-call  VariantControl=(inherit)
  Display : Display
  GetPeriod_ms : $bdroot/GetPeriod_ms  frqP=TRI_frqFreeSys_val
  Write Measurement : CoderSF_BSW_Libs/Calibration & Measurement/Write Measurement  variable_name=TRI_tL500ms  variable_value=0  variable_type=single  numD=1  unitStr=ms  descStr=""
      settings: AttributesFormatString=value:%<variable_value> type:%<variable_type>  SourceProductName=EcoCoder Blocks
  dt : CoderSF_BSW_Libs/Application Base Blocks/dt
      settings: SourceProductName=EcoCoder Blocks
  wires:
  GetPeriod_ms/1 -> Write Measurement/1
  dt/1 -> Display/1
